simulink model "Simulation2024a"  (R2024a)
settings: Solver=ode8  StartTime=0.0  StopTime=0.002  FixedStep=0.00001  RelTol=1e-3
InitFcn:
  | R=120;
  | L=6e-3;
  | C=0.1e-6;
libraries: fl_lib x6, nesl_utility x3
settings Model: LastModifiedBy=Antony

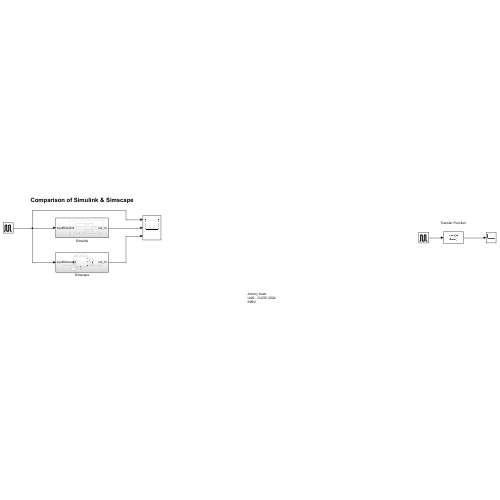
[thumbnail: Simulink's stored preview of the top-level diagram]
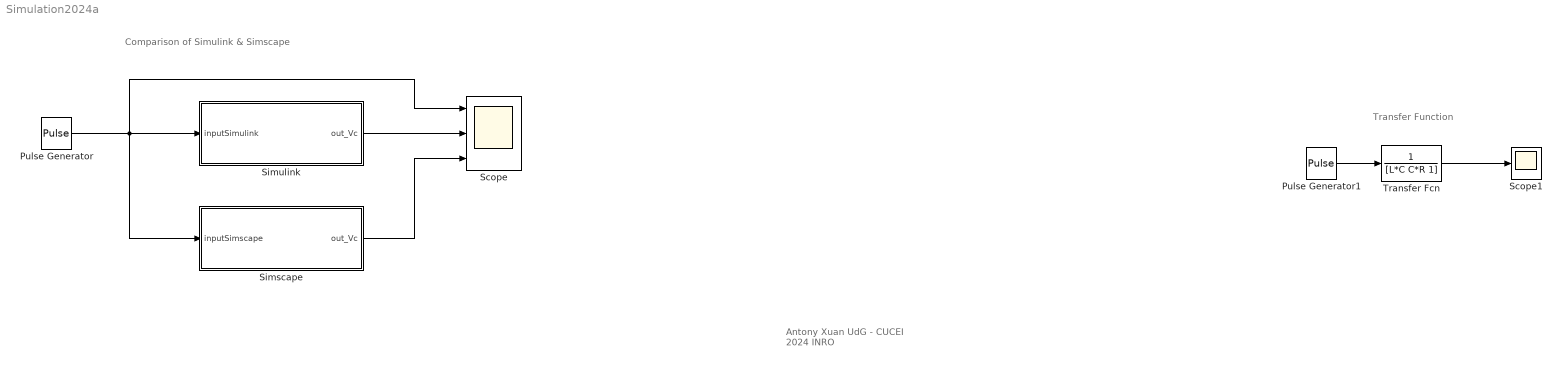
== system Simulation2024a ==
  note: Antony Xuan
      | UdG - CUCEI 2024
      | INRO
  note: Comparison of Simulink & Simscape
  note: Transfer Function
  Pulse Generator : DiscretePulseGenerator  PulseType=Time based  Amplitude=5  Period=0.002  PulseWidth=50
  Pulse Generator1 : DiscretePulseGenerator  PulseType=Time based  Amplitude=5  Period=0.02  PulseWidth=50
  Scope : Scope  NumInputPorts=3
  Scope1 : Scope
  Simscape : Subsystem
  Simulink : Subsystem
  Transfer Fcn : TransferFcn  Denominator=[L*C C*R 1]
  wires:
  Pulse Generator/1 -> Scope/1, Simscape/1(inputSimscape), Simulink/1(inputSimulink)
  Simulink/1(out_Vc) -> Scope/2
  Simscape/1(out_Vc) -> Scope/3
  Pulse Generator1/1 -> Transfer Fcn/1
  Transfer Fcn/1 -> Scope1/1

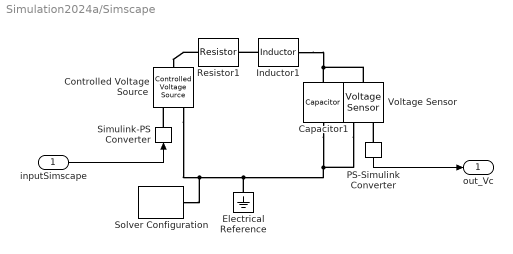
== system Simulation2024a/Simscape ==
  inputSimscape : Inport
  Capacitor1 : fl_lib/Electrical/Electrical Elements/Capacitor  c=C F  r=1e-6 Ohm  g=0 1/Ohm  i_specify=off  i_priority=None  i=0 A  i_nominal_specify=off  i_nominal_value=1  i_nominal_unit=A  v_specify=off  v_priority=None  v=0 V  v_nominal_specify=off  v_nominal_value=1  v_nominal_unit=V  vc_specify=off  vc_priority=High  vc=0 V  vc_nominal_specify=off  vc_nominal_value=1  vc_nominal_unit=V
  Controlled Voltage Source : fl_lib/Electrical/Electrical Sources/Controlled Voltage Source
  Electrical Reference : fl_lib/Electrical/Electrical Elements/Electrical Reference
  Inductor1 : fl_lib/Electrical/Electrical Elements/Inductor  l=L H  r=0 Ohm  g=1e-9 1/Ohm  i_specify=off  i_priority=None  i=0 A  i_nominal_specify=off  i_nominal_value=1  i_nominal_unit=A  v_specify=off  v_priority=None  v=0 V  v_nominal_specify=off  v_nominal_value=1  v_nominal_unit=V  i_L_specify=off  i_L_priority=High  i_L=0 A  i_L_nominal_specify=off  i_L_nominal_value=1  i_L_nominal_unit=A
  PS-Simulink Converter : nesl_utility/PS-Simulink Converter  PhysicalDomain=network_engine_domain  SubClassName=ps_output  LeftPortType=input  RightPortType=output  PseudoPeriodic=off  Frequencies=[]  VectorFormat=inherit  Unit=inherit  AffineConversion=off
  Resistor1 : fl_lib/Electrical/Electrical Elements/Resistor  R=R Ohm  i_specify=off  i_priority=None  i=0 A  i_nominal_specify=off  i_nominal_value=1  i_nominal_unit=A  v_specify=off  v_priority=None  v=0 V  v_nominal_specify=off  v_nominal_value=1  v_nominal_unit=V
  Simulink-PS Converter : nesl_utility/Simulink-PS Converter  PhysicalDomain=network_engine_domain  SubClassName=ps_input  LeftPortType=input  RightPortType=output  PseudoPeriodic=off  Frequencies=[]  NoiseDistribution=none  NoiseParameters=[]  Unit=1  AffineConversion=off  FilteringAndDerivatives=provide  SimscapeFilterOrder=1  InputFilterTimeConstant=0.001  UdotUserProvided=0
  Solver Configuration : nesl_utility/Solver Configuration  PhysicalDomain=network_engine_domain  SubClassName=solver  LeftPortType=input  RightPortType=generic  Tones=[]  Harmonics=[]  SimulateNoise=off  Profile=off  UseLocalSampling=off  EnableSwitchedLinearOptims=on  FrequencyDomain=off  UseCCode=off  RelTol=0.001  AbsTol=0.001  MinStep=1e-09  ToWorkspace=off  RevertToSquareIcSolve=off  NumHomotopyIterations=100  PhasorMode=off  PhasorModeNumHarmonics=1  ConsistencySolver=NEWTON_XTOL_AFTER_FTOL  IndexReductionMethod=DerivativeReplacement  DoDC=off  ResidualTolerance=1e-09  ConsistencyTolSource=GLOBAL  ConsistencyAbsTol=0.001  ConsistencyRelTol=0.001  ConsistencyTolFactor=0.001  UseLocalSolver=off  LocalSolverChoice=NE_BACKWARD_EULER_ADVANCER  ResolveIndetEquations=on  FunctionEvalNumThread=1  LocalSolverSampleTime=0.001  DoFixedCost=off  MaxNonlinIter=3  MaxModeIter=2  ComputeImpulses=off  ImpulseIterations=2  LinearAlgebra=auto  LinearAlgebraNumThread=0  EquationFormulation=NE_TIME_EF  DelaysMemoryBudget=1024  AutomaticFiltering=on  FilteringTimeConstant=0.001  PartitionStorageMethod=AS_NEEDED  PartitionMemoryBudget=1024  PartitionMethod=ROBUST  MultibodyUseLocalSolver=off  MultibodyLocalSolverChoice=ODE1  MultibodyLocalSolverSampleTime=0.001
  Voltage Sensor : fl_lib/Electrical/Electrical Sensors/Voltage Sensor
  out_Vc : Outport
  wires:
  inputSimscape/1 -> Simulink-PS Converter/1
  PS-Simulink Converter/1 -> out_Vc/1
  connections:
  PS-Simulink Converter/LConn1 -- Voltage Sensor/RConn1
  Inductor1/LConn1 -- Resistor1/RConn1
  Simulink-PS Converter/RConn1 -- Controlled Voltage Source/RConn1
  Voltage Sensor/LConn1 -- Capacitor1/LConn1 -- Inductor1/RConn1
  Resistor1/LConn1 -- Controlled Voltage Source/LConn1
  Controlled Voltage Source/RConn2 -- Solver Configuration/RConn1 -- Capacitor1/RConn1 -- Voltage Sensor/RConn2 -- Electrical Reference/LConn1

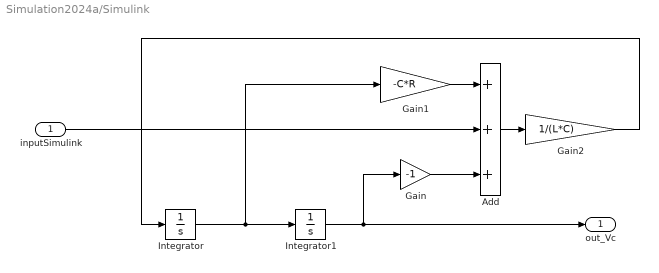
== system Simulation2024a/Simulink ==
  inputSimulink : Inport
  Add : Sum  Inputs=+++
  Gain : Gain  Gain=-1
  Gain1 : Gain  Gain=-C*R
  Gain2 : Gain  Gain=1/(L*C)
  Integrator : Integrator
  Integrator1 : Integrator
  out_Vc : Outport
  wires:
  Gain/1 -> Add/3
  Gain1/1 -> Add/1
  Gain2/1 -> Integrator/1
  Integrator/1 -> Gain1/1, Integrator1/1
  Add/1 -> Gain2/1
  Integrator1/1 -> out_Vc/1, Gain/1
  inputSimulink/1 -> Add/2
